simulink model "SPWM_simulink_deadtime"  (R2014b)
settings: Solver=ode23tb  StartTime=0.0  StopTime=0.05  MaxStep=0.00001  RelTol=1e-3
InitFcn:
  | Fc=5000;
  | f=50;
  | Vdc=700;
undefined symbols (not defined in the file): Ts
libraries: powerlib_extras x3, simulink x1, powerlib x1
settings Model: Creator=Lei  LastModifiedBy=Lei

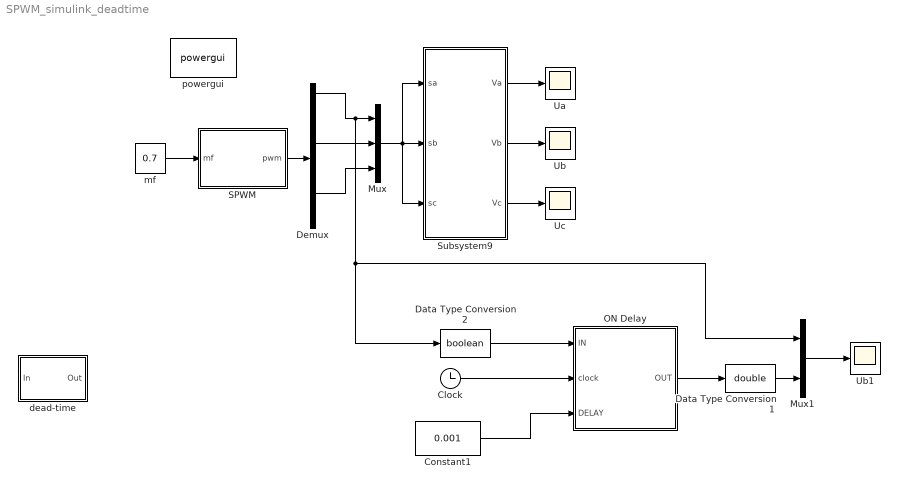
== system SPWM_simulink_deadtime ==
  Clock : Clock
  Constant1 : Constant  Value=0.001
  Data Type Conversion1 : DataTypeConversion  OutDataTypeStr=double  SaturateOnIntegerOverflow=on  RndMeth=Zero
  Data Type Conversion2 : DataTypeConversion  OutDataTypeStr=boolean  SaturateOnIntegerOverflow=on  RndMeth=Zero
  Demux : Demux  Outputs=6
  Mux : Mux  Inputs=3
  Mux1 : Mux  Inputs=2
  ON Delay : Subsystem  TreatAsAtomicUnit=on
  SPWM : Subsystem
  Subsystem9 : Subsystem
  "Ua  " : Scope
      settings: YMin=-500  YMax=500  SaveName=Ua  SampleInput=on
  Ub : Scope
      settings: YMin=-500  YMax=500  SaveName=Ua1  SampleInput=on
  Ub1 : Scope
      settings: TimeRange=0.003608515057113188  YMin=0.8454391891891893  YMax=0.8471283783783784  SaveName=Ua3  SampleInput=on
  Uc : Scope
      settings: YMin=-500  YMax=500  SaveName=Ua2  SampleInput=on
  dead-time : Subsystem
  mf : Constant  Value=0.7
  powergui : powerlib/powergui  Priority=1  SimulationMode=Continuous  SolverType=Tustin/Backward Euler (TBE)  SampleTime=50e-6  frequency=60  SPID=off  DisableSnubberDevices=off  DisableRonSwitches=off  DisableVfSwitches=off  SwTol=0  DisplayEquations=off  Interpol=off  methode=off  Ts=100  frequencyindice=60  Pbase=100e6  ErrMax=1e-4  Iterations=50  UnitsV=kV  UnitsW=MW  FunctionMessages=off  echomessages=off  HookPort=off  EnableUseOfTLC=off  x0status=blocks  RestoreLinks=warning  ResistiveCurrentMeasurement=off  Frange=[0:2:500]  Ylog=off  Xlog=on  ShowGrid=off  save=off  variable=ZData  structure=Ua  ZoomFFT=off  StartTime=0  cycles=1  DisplayStyle=1  fundamental=50  FreqAxis=off  MaxFrequency=9000  frequencyindicesteady=1  RmsSteady=1  display=off
  wires:
  mf/1 -> SPWM/1(mf)
  Subsystem9/1(Va) -> "Ua  "/1
  Subsystem9/2(Vb) -> Ub/1
  Subsystem9/3(Vc) -> Uc/1
  SPWM/1(pwm) -> Demux/1
  Demux/3 -> Mux/2
  Demux/5 -> Mux/3
  Mux/1 -> Subsystem9/1(sa), Subsystem9/3(sc), Subsystem9/2(sb)
  Demux/1 -> Mux1/1, Data Type Conversion2/1, Mux/1
  ON Delay/1(OUT) -> Data Type Conversion1/1
  Constant1/1 -> ON Delay/3(DELAY)
  Clock/1 -> ON Delay/2(clock)
  Mux1/1 -> Ub1/1
  Data Type Conversion2/1 -> ON Delay/1(IN)
  Data Type Conversion1/1 -> Mux1/2

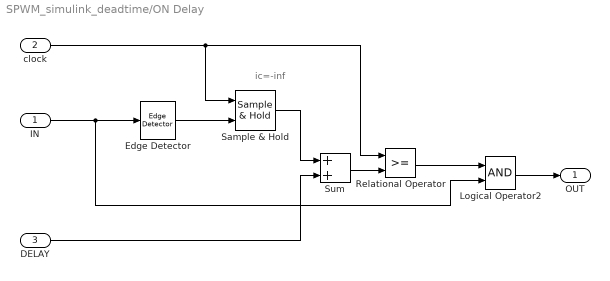
== system SPWM_simulink_deadtime/ON Delay ==
  note: ic=-inf
  IN : Inport
  clock : Inport  Port=2
  DELAY : Inport  Port=3
  Edge Detector : powerlib_extras/Control  Blocks/Edge Detector  model=Rising  ic=0
  Logical Operator2 : Logic
  Relational Operator : RelationalOperator  OutDataTypeStr=boolean  InputSameDT=on
  Sample & Hold : powerlib_extras/Control  Blocks/Sample & Hold  ic=-1e99
  Sum : Sum  SaturateOnIntegerOverflow=on  InputSameDT=on  OutDataTypeStr=Inherit: Same as first input
  OUT : Outport
  wires:
  Sample & Hold/1 -> Sum/1
  Edge Detector/1 -> Sample & Hold/2
  Relational Operator/1 -> Logical Operator2/1
  DELAY/1 -> Sum/2
  Sum/1 -> Relational Operator/2
  clock/1 -> Sample & Hold/1, Relational Operator/1
  IN/1 -> Edge Detector/1, Logical Operator2/2
  Logical Operator2/1 -> OUT/1

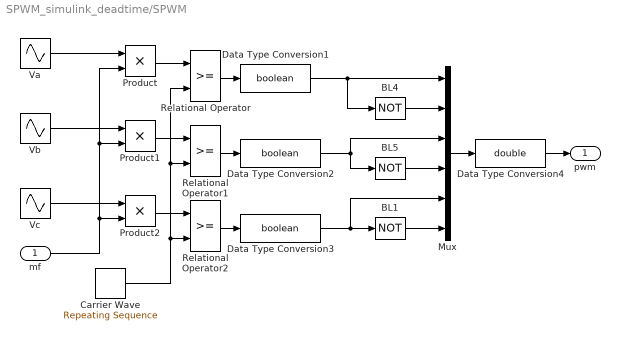
== system SPWM_simulink_deadtime/SPWM ==
  mf : Inport
  BL1 : Logic  Operator=NOT  Inputs=1
  BL4 : Logic  Operator=NOT  Inputs=1
  BL5 : Logic  Operator=NOT  Inputs=1
  Carrier Wave : simulink/Sources/Repeating Sequence  rep_seq_t=[0 1/Fc/4 3/Fc/4 1/Fc]  rep_seq_y=[0 -1 1 0]
  Data Type Conversion1 : DataTypeConversion  OutDataTypeStr=boolean  SaturateOnIntegerOverflow=on  RndMeth=Zero
  Data Type Conversion2 : DataTypeConversion  OutDataTypeStr=boolean  SaturateOnIntegerOverflow=on  RndMeth=Zero
  Data Type Conversion3 : DataTypeConversion  OutDataTypeStr=boolean  SaturateOnIntegerOverflow=on  RndMeth=Zero
  Data Type Conversion4 : DataTypeConversion  OutDataTypeStr=double  SaturateOnIntegerOverflow=on  RndMeth=Zero
  Mux : Mux  Inputs=6
  Product : Product
  Product1 : Product
  Product2 : Product
  Relational Operator : RelationalOperator  InputSameDT=on
  Relational Operator1 : RelationalOperator  InputSameDT=on
  Relational Operator2 : RelationalOperator  InputSameDT=on
  Va : Sin  Frequency=2*pi*f  SampleTime=0
  Vb : Sin  Frequency=2*pi*f  Phase=-2*pi/3  SampleTime=0
  Vc : Sin  Frequency=2*pi*f  Phase=2*pi/3  SampleTime=0
  pwm : Outport
  wires:
  Carrier Wave/1 -> Relational Operator1/2, Relational Operator/2, Relational Operator2/2
  Data Type Conversion1/1 -> Mux/1, BL4/1
  Relational Operator/1 -> Data Type Conversion1/1
  Data Type Conversion2/1 -> BL5/1, Mux/3
  Relational Operator1/1 -> Data Type Conversion2/1
  BL4/1 -> Mux/2
  Relational Operator2/1 -> Data Type Conversion3/1
  BL5/1 -> Mux/4
  BL1/1 -> Mux/6
  Data Type Conversion3/1 -> Mux/5, BL1/1
  Mux/1 -> Data Type Conversion4/1
  Product2/1 -> Relational Operator2/1
  Product1/1 -> Relational Operator1/1
  Vb/1 -> Product1/1
  Va/1 -> Product/1
  mf/1 -> Product2/2, Product1/2, Product/2
  Product/1 -> Relational Operator/1
  Vc/1 -> Product2/1
  Data Type Conversion4/1 -> pwm/1

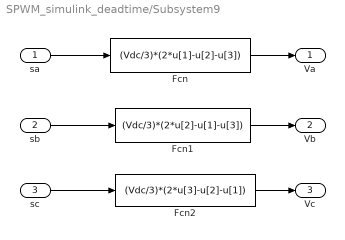
== system SPWM_simulink_deadtime/Subsystem9 ==
  sa : Inport
  sb : Inport  Port=2
  sc : Inport  Port=3
  Fcn : Fcn  Expr=(Vdc/3)*(2*u[1]-u[2]-u[3])
  Fcn1 : Fcn  Expr=(Vdc/3)*(2*u[2]-u[1]-u[3])
  Fcn2 : Fcn  Expr=(Vdc/3)*(2*u[3]-u[2]-u[1])
  Va : Outport
  Vb : Outport  Port=2
  Vc : Outport  Port=3
  wires:
  Fcn/1 -> Va/1
  Fcn1/1 -> Vb/1
  Fcn2/1 -> Vc/1
  sa/1 -> Fcn/1
  sb/1 -> Fcn1/1
  sc/1 -> Fcn2/1

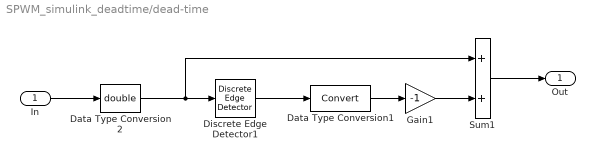
== system SPWM_simulink_deadtime/dead-time ==
  In : Inport
  Data Type Conversion1 : DataTypeConversion
  Data Type Conversion2 : DataTypeConversion  OutDataTypeStr=double
  Discrete Edge Detector1 : powerlib_extras/Discrete  Control Blocks/Discrete Edge Detector  model=Rising  ic=0.001  Ts=5*Ts
  Gain1 : Gain  Gain=-1
  Sum1 : Sum
  Out : Outport
  wires:
  Discrete Edge Detector1/1 -> Data Type Conversion1/1
  Data Type Conversion1/1 -> Gain1/1
  Gain1/1 -> Sum1/2
  In/1 -> Data Type Conversion2/1
  Sum1/1 -> Out/1
  Data Type Conversion2/1 -> Sum1/1, Discrete Edge Detector1/1
